simulink model "ieee9"  (R2021a)
settings: Solver=VariableStepAuto  StartTime=0.0  StopTime=10.0  RelTol=1e-3
values from neighbouring files (symbols this model uses):
  k5 = rand()    [data_generator.m]
  k6 = rand()    [data_generator.m]
  k8 = rand()    [data_generator.m]
libraries: spsThreePhaseVIMeasurementLib x9, spsLoadFlowBusLib x9, spsThreePhaseSeriesRLCBranchLib x6, spsThreePhaseSourceLib x3, spsThreePhaseParallelRLCLoadLib x3, spsThreePhaseTransformerTwoWindingsLib x3, spspowerguiLib x1
settings Model: Creator=Eduardo Trabajo  LastModifiedBy=Eduardo Trabajo
settings DebuggingCC: UnconnectedInputMsg=none  UnconnectedOutputMsg=none  UnconnectedLineMsg=none

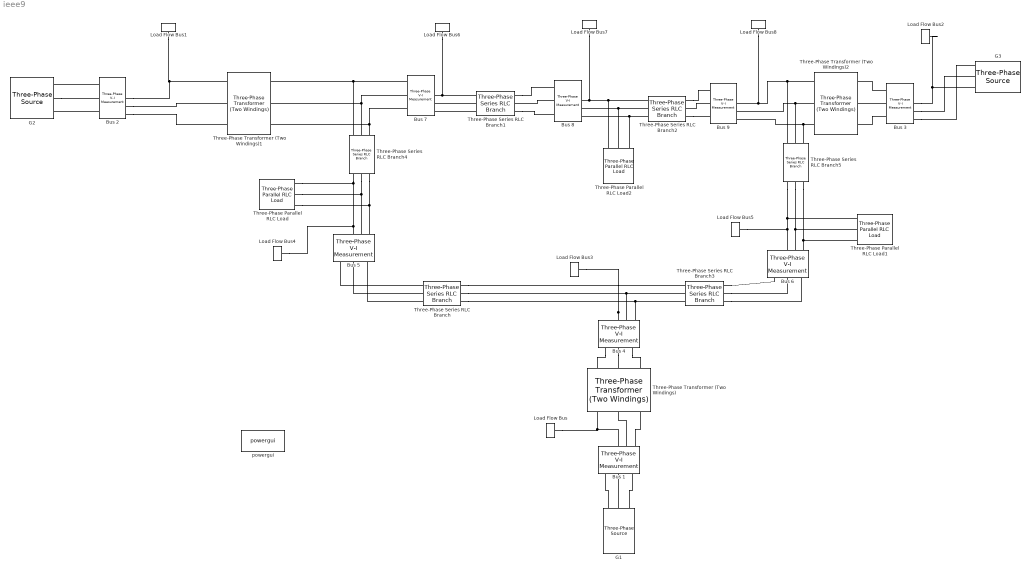
== system ieee9 ==
  Bus {1..9} (9 alike) : spsThreePhaseVIMeasurementLib/Three-Phase V-I Measurement  VoltageMeasurement=phase-to-ground  SetLabelV=off  LabelV=Vabc  Vpu=off  VpuLL=off  CurrentMeasurement=yes  SetLabelI=off  LabelI=Iabc  Ipu=off  Pbase=100e6  Vbase=500e3  OutputType=Complex  PhasorSimulation=off  PSBequivalent=0
  G1 : spsThreePhaseSourceLib/Three-Phase Source  InternalConnection=Yg  VoltagePhases=off  Voltage=(24000)*1  PhaseAngle=0  Voltage_phases=[25e3 25e3 25e3]/sqrt(3)  PhaseAngles_phases=[0 -120 +120]  Frequency=60  NonIdealSource=off  SpecifyImpedance=off  Resistance=0.8929  Inductance=16.58e-3  ShortCircuitLevel=100e6  BaseVoltage=24e3  XRratio=7  BusType=swing  Pref=10e3  Qref=0  Prefabc=[10e3, 10e3, 10e3]  Qrefabc=[0, 0, 0]  Qmin=-inf  Qmax=inf
  G2 : spsThreePhaseSourceLib/Three-Phase Source  InternalConnection=Yg  VoltagePhases=off  Voltage=(18000)*0.949719  PhaseAngle=18.4022  Voltage_phases=[25e3 25e3 25e3]/sqrt(3)  PhaseAngles_phases=[0 -120 +120]  Frequency=60  NonIdealSource=off  SpecifyImpedance=off  Resistance=0.8929  Inductance=16.58e-3  ShortCircuitLevel=100e6  BaseVoltage=18e3  XRratio=7  BusType=PQ  Pref=163e6  Qref=4.9e6  Prefabc=[10e3, 10e3, 10e3]  Qrefabc=[0, 0, 0]  Qmin=-inf  Qmax=inf
  G3 : spsThreePhaseSourceLib/Three-Phase Source  InternalConnection=Yg  VoltagePhases=off  Voltage=(13800)*0.954898  PhaseAngle=13.6753  Voltage_phases=[25e3 25e3 25e3]/sqrt(3)  PhaseAngles_phases=[0 -120 +120]  Frequency=60  NonIdealSource=off  SpecifyImpedance=off  Resistance=0.8929  Inductance=16.58e-3  ShortCircuitLevel=100e6  BaseVoltage=13.8e3  XRratio=7  BusType=PQ  Pref=85e6  Qref=11.45e6  Prefabc=[10e3, 10e3, 10e3]  Qrefabc=[0, 0, 0]  Qmin=-inf  Qmax=inf
  Load Flow Bus : spsLoadFlowBusLib/Load Flow Bus  LConnTagsString=a  Phases=single  Connectors=on one side  ID=BUS_1  Vbase=24e3  Vref=1  Vangle=0  VLF=1  VLFb=1  VLFc=1  angleLF=0  angleLFb=0  angleLFc=0
      settings: SourceProductBaseCode=PS
  Load Flow Bus1 : spsLoadFlowBusLib/Load Flow Bus  LConnTagsString=a  Phases=single  Connectors=on one side  ID=BUS_2  Vbase=18e3  Vref=1  Vangle=0  VLF=0.9497  VLFb=1  VLFc=1  angleLF=18.4  angleLFb=0  angleLFc=0
      settings: SourceProductBaseCode=PS
  Load Flow Bus2 : spsLoadFlowBusLib/Load Flow Bus  LConnTagsString=a  Phases=single  Connectors=on one side  ID=BUS_3  Vbase=13.8e3  Vref=1  Vangle=0  VLF=0.9549  VLFb=1  VLFc=1  angleLF=13.68  angleLFb=0  angleLFc=0
      settings: SourceProductBaseCode=PS
  Load Flow Bus3 : spsLoadFlowBusLib/Load Flow Bus  LConnTagsString=a  Phases=single  Connectors=on one side  ID=BUS_4  Vbase=230e3  Vref=1  Vangle=0  VLF=0.9803  VLFb=1  VLFc=1  angleLF=1.426  angleLFb=0  angleLFc=0
      settings: SourceProductBaseCode=PS
  Load Flow Bus4 : spsLoadFlowBusLib/Load Flow Bus  LConnTagsString=a  Phases=single  Connectors=on one side  ID=BUS_5  Vbase=230e3  Vref=1  Vangle=0  VLF=0.9585  VLFb=1  VLFc=1  angleLF=6.177  angleLFb=0  angleLFc=0
      settings: SourceProductBaseCode=PS
  Load Flow Bus5 : spsLoadFlowBusLib/Load Flow Bus  LConnTagsString=a  Phases=single  Connectors=on one side  ID=BUS_6  Vbase=230e3  Vref=1  Vangle=0  VLF=0.943  VLFb=1  VLFc=1  angleLF=2.984  angleLFb=0  angleLFc=0
      settings: SourceProductBaseCode=PS
  Load Flow Bus6 : spsLoadFlowBusLib/Load Flow Bus  LConnTagsString=a  Phases=single  Connectors=on one side  ID=BUS_7  Vbase=230e3  Vref=1  Vangle=0  VLF=0.9494  VLFb=1  VLFc=1  angleLF=15.81  angleLFb=0  angleLFc=0
      settings: SourceProductBaseCode=PS
  Load Flow Bus7 : spsLoadFlowBusLib/Load Flow Bus  LConnTagsString=a  Phases=single  Connectors=on one side  ID=BUS_8  Vbase=230e3  Vref=1  Vangle=0  VLF=0.9347  VLFb=1  VLFc=1  angleLF=12.53  angleLFb=0  angleLFc=0
      settings: SourceProductBaseCode=PS
  Load Flow Bus8 : spsLoadFlowBusLib/Load Flow Bus  LConnTagsString=a  Phases=single  Connectors=on one side  ID=BUS_9  Vbase=230e3  Vref=1  Vangle=0  VLF=0.9523  VLFb=1  VLFc=1  angleLF=12.42  angleLFb=0  angleLFc=0
      settings: SourceProductBaseCode=PS
  Three-Phase Parallel RLC Load : spsThreePhaseParallelRLCLoadLib/Three-Phase Parallel RLC Load  LConnTagsString=A|B|C  Configuration=Y (grounded)  NominalVoltage=230e3  Vabc=[1e3 1e3 1e3]  Vabcp=[1e3 1e3 1e3]  NominalFrequency=60  UnbalancedPower=off  ActivePower=k5*125e6  InductivePower=k5*50e6  CapacitivePower=0  Pabc=[10e3 9e3 11e3]  QLabc=[100 90 110]  QCabc=[100 90 110]  Pabcp=[10e3 9e3 11e3]  QLabcp=[100 90 110]  QCabcp=[100 90 110]  Measurements=None  LoadType=constant Z
  Three-Phase Parallel RLC Load1 : spsThreePhaseParallelRLCLoadLib/Three-Phase Parallel RLC Load  LConnTagsString=A|B|C  Configuration=Y (grounded)  NominalVoltage=230e3  Vabc=[1e3 1e3 1e3]  Vabcp=[1e3 1e3 1e3]  NominalFrequency=60  UnbalancedPower=off  ActivePower=k6*90e6  InductivePower=k6*30e6  CapacitivePower=0  Pabc=[10e3 9e3 11e3]  QLabc=[100 90 110]  QCabc=[100 90 110]  Pabcp=[10e3 9e3 11e3]  QLabcp=[100 90 110]  QCabcp=[100 90 110]  Measurements=None  LoadType=constant Z
  Three-Phase Parallel RLC Load2 : spsThreePhaseParallelRLCLoadLib/Three-Phase Parallel RLC Load  LConnTagsString=A|B|C  Configuration=Y (grounded)  NominalVoltage=230e3  Vabc=[1e3 1e3 1e3]  Vabcp=[1e3 1e3 1e3]  NominalFrequency=60  UnbalancedPower=off  ActivePower=k8*100e6  InductivePower=k8*35e6  CapacitivePower=0  Pabc=[10e3 9e3 11e3]  QLabc=[100 90 110]  QCabc=[100 90 110]  Pabcp=[10e3 9e3 11e3]  QLabcp=[100 90 110]  QCabcp=[100 90 110]  Measurements=None  LoadType=constant Z
  Three-Phase Series RLC Branch : spsThreePhaseSeriesRLCBranchLib/Three-Phase Series RLC Branch  LConnTagsString=A|B|C  RConnTagsString=A|B|C  BranchType=RL  Resistance=89.93*0.0588  Inductance=1.33e-3 *89.93  Capacitance=9.81e-9 *89.93  Measurements=None
  Three-Phase Series RLC Branch1 : spsThreePhaseSeriesRLCBranchLib/Three-Phase Series RLC Branch  LConnTagsString=A|B|C  RConnTagsString=A|B|C  BranchType=RL  Resistance=76.176*5.9e-2  Inductance=76.176*1.33e-3  Capacitance=76.176*9.81e-9  Measurements=None
  Three-Phase Series RLC Branch2 : spsThreePhaseSeriesRLCBranchLib/Three-Phase Series RLC Branch  LConnTagsString=A|B|C  RConnTagsString=A|B|C  BranchType=RL  Resistance=106.646*5.90e-2  Inductance=106.646*1.33e-3  Capacitance=106.646*9.83e-9  Measurements=None
  Three-Phase Series RLC Branch3 : spsThreePhaseSeriesRLCBranchLib/Three-Phase Series RLC Branch  LConnTagsString=A|B|C  RConnTagsString=A|B|C  BranchType=RL  Resistance=97.336*9.24e-2  Inductance=97.336*1.33e-3  Capacitance=97.336*8.14e-9  Measurements=None
  Three-Phase Series RLC Branch4 : spsThreePhaseSeriesRLCBranchLib/Three-Phase Series RLC Branch  LConnTagsString=A|B|C  RConnTagsString=A|B|C  BranchType=RL  Resistance=170.336*9.94e-2  Inductance=170.336*1.33e-3  Capacitance=170.336*9.01e-9  Measurements=None
  Three-Phase Series RLC Branch5 : spsThreePhaseSeriesRLCBranchLib/Three-Phase Series RLC Branch  LConnTagsString=A|B|C  RConnTagsString=A|B|C  BranchType=RL  Resistance=179.86*1.15e-1  Inductance=179.86*1.33e-3  Capacitance=179.86*9.98e-9  Measurements=None
  Three-Phase Transformer (Two Windings) : spsThreePhaseTransformerTwoWindingsLib/Three-Phase Transformer (Two Windings)  Winding1Connection=Yg  Winding2Connection=Yg  CoreType=Three single-phase transformers  SetSaturation=off  Hysteresis=off  DataFile='hysteresis'  SetInitialFlux=off  Measurements=None  UNITS=pu  NominalPower=[ 250e6 , 60 ]  Winding1=[ 24e3 , 1e-10, 2.88e-2 ]  Winding2=[ 230e3 , 1e-10 , 2.88e-2 ]  Rm=5000  Lm=5000  L0=0.5  Saturation=[ 0,0 ; 0.0024,1.2 ; 1.0,1.52 ]  InitialFluxes=[ 0.8 , -0.8 , 0.7 ]  BreakLoop=off  DiscreteSolver=Trapezoidal iterative  DataType=off  TransfoNumber=1
  Three-Phase Transformer (Two Windings)1 : spsThreePhaseTransformerTwoWindingsLib/Three-Phase Transformer (Two Windings)  Winding1Connection=Yg  Winding2Connection=Yg  CoreType=Three single-phase transformers  SetSaturation=off  Hysteresis=off  DataFile='hysteresis'  SetInitialFlux=off  Measurements=None  UNITS=pu  NominalPower=[ 250e6 , 60 ]  Winding1=[ 18e3 , 1e-10 , 3.13e-2 ]  Winding2=[ 230e3 , 1e-10 , 3.13e-2 ]  Rm=5000  Lm=5000  L0=0.5  Saturation=[ 0,0 ; 0.0024,1.2 ; 1.0,1.52 ]  InitialFluxes=[ 0.8 , -0.8 , 0.7 ]  BreakLoop=off  DiscreteSolver=Trapezoidal iterative  DataType=off  TransfoNumber=1
  Three-Phase Transformer (Two Windings)2 : spsThreePhaseTransformerTwoWindingsLib/Three-Phase Transformer (Two Windings)  Winding1Connection=Yg  Winding2Connection=Yg  CoreType=Three single-phase transformers  SetSaturation=off  Hysteresis=off  DataFile='hysteresis'  SetInitialFlux=off  Measurements=None  UNITS=pu  NominalPower=[ 250e6 , 60 ]  Winding1=[ 230e3 , 1e-10 , 2.93e-2 ]  Winding2=[ 13.8e3 , 1e-10 , 2.93e-2 ]  Rm=5000  Lm=5000  L0=0.5  Saturation=[ 0,0 ; 0.0024,1.2 ; 1.0,1.52 ]  InitialFluxes=[ 0.8 , -0.8 , 0.7 ]  BreakLoop=off  DiscreteSolver=Trapezoidal iterative  DataType=off  TransfoNumber=1
  powergui : spspowerguiLib/powergui  Priority=1  SimulationMode=Continuous  SampleTime=50e-6  frequency=60  Iterations=50  frequencyindice=60  Pbase=100e6  ErrMax=1e-4  UnitsV=kV  UnitsW=MW  buscounter=0  FunctionMessages=off  echomessages=off  EnableUseOfTLC=off  CurrentSourceSwitches=off  DisableSnubberDevices=off  DisableRonSwitches=off  DisableVfSwitches=off  DisplayEquations=off  AutomaticDiscreteSolvers=off  SolverType=Tustin/Backward Euler (TBE)  Interpol=off  ExternalGateDelay=off  methode=off  Ts=100  x0status=blocks  SPID=on  SwTol=0  HookPort=off  NonlinearTolerance=1e-4  nMaxIteration=100  ContinueOnMaxIteration=off  RestoreLinks=warning  ResistiveCurrentMeasurement=off  Frange=[0:2:500]  Ylog=off  Xlog=on  ShowGrid=off  save=off  variable=ZData  structure=0  ZoomFFT=off  StartTime=0.0  cycles=1  DisplayStyle=1  fundamental=60  FreqAxis=off  MaxFrequency=1000  frequencyindicesteady=1  RmsSteady=1  display=off
  connections:
  Bus 2/LConn1 -- G2/RConn1
  G2/RConn2 -- Bus 2/LConn2
  Bus 2/LConn3 -- G2/RConn3
  Bus 2/RConn1 -- Load Flow Bus1/LConn1 -- Three-Phase Transformer (Two Windings)1/LConn1
  Bus 2/RConn2 -- Three-Phase Transformer (Two Windings)1/LConn2
  Bus 2/RConn3 -- Three-Phase Transformer (Two Windings)1/LConn3
  Bus 7/LConn1 -- Three-Phase Series RLC Branch4/RConn1 -- Three-Phase Transformer (Two Windings)1/RConn1
  Bus 7/LConn2 -- Three-Phase Series RLC Branch4/RConn2 -- Three-Phase Transformer (Two Windings)1/RConn2
  Bus 7/LConn3 -- Three-Phase Series RLC Branch4/RConn3 -- Three-Phase Transformer (Two Windings)1/RConn3
  Three-Phase Series RLC Branch1/LConn1 -- Load Flow Bus6/LConn1 -- Bus 7/RConn1
  Three-Phase Series RLC Branch1/LConn2 -- Bus 7/RConn2
  Three-Phase Series RLC Branch1/LConn3 -- Bus 7/RConn3
  Three-Phase Series RLC Branch2/LConn1 -- Three-Phase Parallel RLC Load2/LConn1 -- Load Flow Bus7/LConn1 -- Bus 8/RConn1
  Three-Phase Series RLC Branch2/LConn2 -- Three-Phase Parallel RLC Load2/LConn2 -- Bus 8/RConn2
  Three-Phase Series RLC Branch2/LConn3 -- Three-Phase Parallel RLC Load2/LConn3 -- Bus 8/RConn3
  Three-Phase Series RLC Branch1/RConn1 -- Bus 8/LConn1
  Bus 8/LConn2 -- Three-Phase Series RLC Branch1/RConn2
  Three-Phase Series RLC Branch1/RConn3 -- Bus 8/LConn3
  Three-Phase Series RLC Branch2/RConn1 -- Bus 9/LConn1
  Bus 9/LConn2 -- Three-Phase Series RLC Branch2/RConn2
  Three-Phase Series RLC Branch2/RConn3 -- Bus 9/LConn3
  Bus 4/RConn1 -- Three-Phase Series RLC Branch/RConn1 -- Three-Phase Series RLC Branch3/RConn1 -- Load Flow Bus3/LConn1
  Three-Phase Series RLC Branch3/RConn2 -- Three-Phase Series RLC Branch/RConn2 -- Bus 4/RConn2
  Three-Phase Series RLC Branch3/RConn3 -- Three-Phase Series RLC Branch/RConn3 -- Bus 4/RConn3
  Three-Phase Series RLC Branch/LConn1 -- Bus 5/LConn1
  Three-Phase Series RLC Branch/LConn2 -- Bus 5/LConn2
  Three-Phase Series RLC Branch/LConn3 -- Bus 5/LConn3
  Three-Phase Series RLC Branch3/LConn1 -- Bus 6/LConn1
  Three-Phase Series RLC Branch3/LConn2 -- Bus 6/LConn2
  Three-Phase Series RLC Branch3/LConn3 -- Bus 6/LConn3
  Three-Phase Transformer (Two Windings)2/LConn1 -- Three-Phase Series RLC Branch5/RConn1 -- Bus 9/RConn1 -- Load Flow Bus8/LConn1
  Three-Phase Transformer (Two Windings)2/LConn2 -- Three-Phase Series RLC Branch5/RConn2 -- Bus 9/RConn2
  Three-Phase Transformer (Two Windings)2/LConn3 -- Three-Phase Series RLC Branch5/RConn3 -- Bus 9/RConn3
  Bus 3/LConn1 -- Three-Phase Transformer (Two Windings)2/RConn1
  Bus 3/LConn2 -- Three-Phase Transformer (Two Windings)2/RConn2
  Bus 3/LConn3 -- Three-Phase Transformer (Two Windings)2/RConn3
  Bus 3/RConn3 -- G3/RConn3
  Bus 3/RConn2 -- G3/RConn2
  Bus 3/RConn1 -- G3/RConn1 -- Load Flow Bus2/LConn1
  Bus 4/LConn1 -- Three-Phase Transformer (Two Windings)/RConn1
  Bus 4/LConn2 -- Three-Phase Transformer (Two Windings)/RConn2
  Bus 4/LConn3 -- Three-Phase Transformer (Two Windings)/RConn3
  Bus 1/RConn1 -- Load Flow Bus/LConn1 -- Three-Phase Transformer (Two Windings)/LConn1
  Bus 1/RConn2 -- Three-Phase Transformer (Two Windings)/LConn2
  Bus 1/RConn3 -- Three-Phase Transformer (Two Windings)/LConn3
  G1/RConn1 -- Bus 1/LConn1
  G1/RConn2 -- Bus 1/LConn2
  G1/RConn3 -- Bus 1/LConn3
  Three-Phase Series RLC Branch4/LConn1 -- Three-Phase Parallel RLC Load/LConn1 -- Load Flow Bus4/LConn1 -- Bus 5/RConn1
  Three-Phase Series RLC Branch4/LConn2 -- Three-Phase Parallel RLC Load/LConn2 -- Bus 5/RConn2
  Three-Phase Series RLC Branch4/LConn3 -- Three-Phase Parallel RLC Load/LConn3 -- Bus 5/RConn3
  Three-Phase Series RLC Branch5/LConn1 -- Three-Phase Parallel RLC Load1/LConn1 -- Load Flow Bus5/LConn1 -- Bus 6/RConn1
  Three-Phase Series RLC Branch5/LConn2 -- Three-Phase Parallel RLC Load1/LConn2 -- Bus 6/RConn2
  Three-Phase Series RLC Branch5/LConn3 -- Three-Phase Parallel RLC Load1/LConn3 -- Bus 6/RConn3
